simulink model "PowerSupplySimulation3"  (Simulink 8.6)
settings: Solver=VariableStepAuto  StartTime=0.0  StopTime=360e-6  RelTol=1e-3
values from neighbouring files (symbols this model uses):
  Ac = 1/(evalfr(G_ss, wcross)*evalfr(Gc1, wcross)*evalfr(Gc2, wcross))    [CurrentSourceController.m]    (also in VoltageSourceController.m)
  c2_val = 0.1e-6    (= 1e-07)    [VoltageSourceController.m]
  l1_val = 480e-8    (= 4.8e-06)    [CurrentSourceController.m]
  l2_val = 0.01e-6    (= 1e-08)    [VoltageSourceController.m]
  r_val = 1    [CurrentSourceController.m]
  rc2_val = 0.0001    [VoltageSourceController.m]
  rl1_val = 0.0002    [CurrentSourceController.m]
  rl2_val = 0.0001    [VoltageSourceController.m]
  Vd_val = 100    [CurrentSourceController.m]    (also in VoltageSourceController.m)
undefined symbols (not defined in the file or in its folder): den_c1, den_c2, num_c1, num_c2
libraries: powerlib x31, powerlib_meascontrol x2
settings Model: Creator=Akshay  LastModifiedBy=Akshay
settings SolverCC: ZeroCrossAlgorithm=Adaptive
settings DataIOCC: SaveFormat=Dataset  SignalLoggingSaveFormat=Dataset
settings OptimizationCC: ExpressionDepthLimit=128
settings DebuggingCC: UnderspecifiedInitializationDetection=Simplified  MergeDetectMultiDrivingBlocksExec=error  SolverPrmCheckMsg=none  FcnCallInpInsideContextMsg=EnableAllAsError  StateNameClashWarn=none
settings HardwareCC: ProdBitPerPointer=64  ProdLargestAtomicFloat=Float  ProdIntDivRoundTo=Zero  ProdEndianess=LittleEndian  ProdWordSize=64  ProdHWDeviceType=Intel->x86-64 (Windows64)
settings GRTTargetCC: GeneratePreprocessorConditionals=Use local settings  CombineOutputUpdateFcns=on  GRTInterface=off
settings ConfigComp: CovModelRefEnable=off

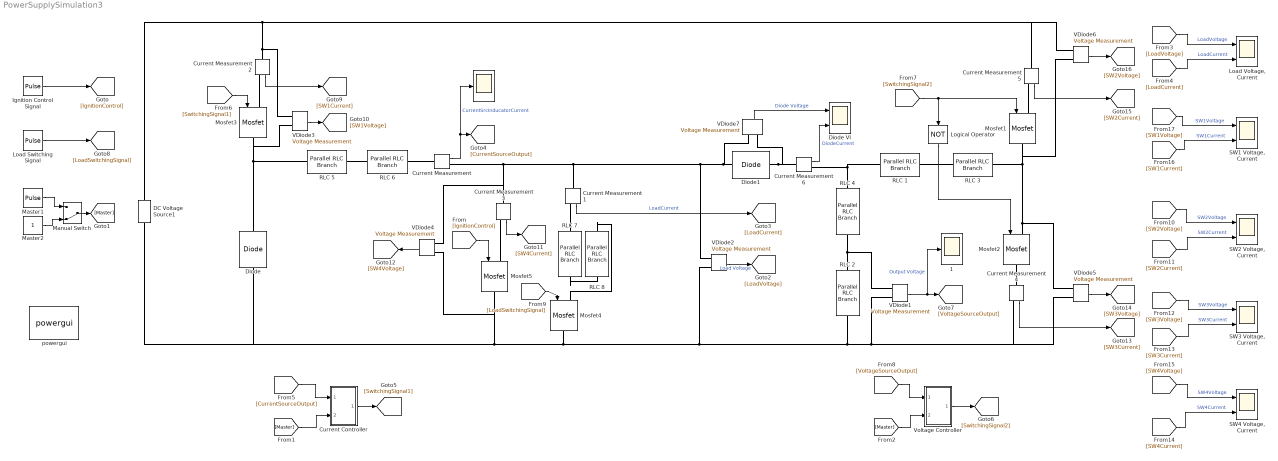
== system PowerSupplySimulation3 ==
  " " : Scope
  " 1" : Scope
  " RLC 1" : powerlib/Elements/Parallel RLC Branch  LConnTagsString=a  RConnTagsString=__new0  BranchType=R  Resistance=rl2_val  Inductance=5e-6  SetiL0=off  InitialCurrent=0  Capacitance=0.3e-6  Setx0=off  InitialVoltage=0  Measurements=None
  " RLC 2" : powerlib/Elements/Parallel RLC Branch  LConnTagsString=a  RConnTagsString=__new0  BranchType=C  Resistance=1  Inductance=1e-3  SetiL0=off  InitialCurrent=0  Capacitance=c2_val  Setx0=off  InitialVoltage=50  Measurements=None
  " RLC 3" : powerlib/Elements/Parallel RLC Branch  LConnTagsString=a  RConnTagsString=__new0  BranchType=L  Resistance=50  Inductance=l2_val  SetiL0=off  InitialCurrent=0  Capacitance=0.3e-6  Setx0=off  InitialVoltage=0  Measurements=None
  " RLC 4" : powerlib/Elements/Parallel RLC Branch  LConnTagsString=a  RConnTagsString=__new0  BranchType=R  Resistance=rc2_val  Inductance=1e-3  SetiL0=off  InitialCurrent=0  Capacitance=0.1e-6  Setx0=off  InitialVoltage=0  Measurements=None
  " RLC 5" : powerlib/Elements/Parallel RLC Branch  LConnTagsString=a  RConnTagsString=__new0  BranchType=R  Resistance=rl1_val  Inductance=5e-6  SetiL0=off  InitialCurrent=0  Capacitance=0.3e-6  Setx0=off  InitialVoltage=0  Measurements=None
  " RLC 6" : powerlib/Elements/Parallel RLC Branch  LConnTagsString=a  RConnTagsString=__new0  BranchType=L  Resistance=50  Inductance=l1_val  SetiL0=off  InitialCurrent=100  Capacitance=0.3e-6  Setx0=off  InitialVoltage=0  Measurements=None
  " RLC 7" : powerlib/Elements/Parallel RLC Branch  LConnTagsString=a  RConnTagsString=__new0  BranchType=R  Resistance=r_val  Inductance=1e-3  SetiL0=off  InitialCurrent=0  Capacitance=0.1e-6  Setx0=off  InitialVoltage=0  Measurements=None
  " RLC 8" : powerlib/Elements/Parallel RLC Branch  LConnTagsString=a  RConnTagsString=__new0  BranchType=L  Resistance=r_val  Inductance=15e-6  SetiL0=off  InitialCurrent=0  Capacitance=0.1e-6  Setx0=off  InitialVoltage=0  Measurements=None
  Current Measurement{,1..6} (7 alike) : powerlib/Measurements/Current Measurement  PhasorSimulation=off  OutputType=Complex  PSBequivalent=0
  Current Controller : Subsystem
  DC Voltage Source1 : powerlib/Electrical Sources/DC Voltage Source  Amplitude=Vd_val  Measurements=Voltage
  Diode : powerlib/Power Electronics/Diode  Ron=0.001  Lon=0  Vf=0.8  IC=0  UseSnubber=off  Rs=500  Cs=250e-9  Measurements=off
  Diode VI : Scope  NumInputPorts=2
  Diode1 : powerlib/Power Electronics/Diode  Ron=0.001  Lon=0  Vf=0.8  IC=0  UseSnubber=off  Rs=500  Cs=250e-9  Measurements=off
  Ignition Control Signal : DiscretePulseGenerator  PulseType=Time based  Period=180e-6  PulseWidth=94  PhaseDelay=6*1.8e-6
  Load Switching Signal : DiscretePulseGenerator  PulseType=Time based  Period=180e-6  PulseWidth=5  PhaseDelay=1.8e-6
  "Load Voltage, Current" : Scope  NumInputPorts=2
  Logical Operator : Logic  Operator=NOT  AllPortsSameDT=off  OutDataTypeStr=boolean
  Manual Switch : ManualSwitch  CurrentSetting=0
  Master1 : DiscretePulseGenerator  PulseType=Time based  Period=180e-6  PulseWidth=6
  Master2 : Constant
  Mosfet{1..5} (5 alike) : powerlib/Power Electronics/Mosfet  Ron=0.00001  Lon=0  Rd=0.0000000000001  Vfd=0  IC=0  Rs=1e5  Cs=inf  Measurements=off
  "SW1 Voltage, Current" : Scope  NumInputPorts=2
  "SW2 Voltage, Current" : Scope  NumInputPorts=2
  "SW3 Voltage, Current" : Scope  NumInputPorts=2
  "SW4 Voltage, Current" : Scope  NumInputPorts=2
  VDiode{1..7} (7 alike) : powerlib/Measurements/Voltage Measurement  PhasorSimulation=off  OutputType=Complex  PSBequivalent=0
  Voltage Controller : Subsystem
  powergui : powerlib/powergui  Priority=1  SimulationMode=Continuous  SolverType=Backward Euler  SampleTime=5e-07  frequency=60  SPID=on  DisableSnubberDevices=off  DisableRonSwitches=off  DisableVfSwitches=off  SwTol=0  DisplayEquations=off  Interpol=off  ExternalGateDelay=off  methode=off  Ts=0  FunctionMessages=off  echomessages=off  HookPort=off  EnableUseOfTLC=off  x0status=zero  frequencyindice=0  Pbase=100e6  ErrMax=1e-4  Iterations=50  UnitsV=kV  UnitsW=MW  buscounter=0  RestoreLinks=warning  ResistiveCurrentMeasurement=off  Frange=[0:2:500]  Ylog=off  Xlog=on  ShowGrid=off  save=off  variable=ZData  structure=ScopeData  ZoomFFT=off  StartTime=0.0  cycles=5  DisplayStyle=2  fundamental=50  FreqAxis=off  MaxFrequency=50000  frequencyindicesteady=1  RmsSteady=1  display=off
  wires:
  Logical Operator/1 -> Mosfet2/1
  VDiode1/1 -> " 1"/1, [VoltageSourceOutput]  "Output Voltage"
  Ignition Control Signal/1 -> [IgnitionControl]
  [IgnitionControl] -> Mosfet5/1
  VDiode2/1 -> [LoadVoltage]  "Load Voltage"
  Current Measurement1/1 -> [LoadCurrent]  "LoadCurrent"
  [LoadVoltage] -> "Load Voltage, Current"/1  "LoadVoltage"
  [LoadCurrent] -> "Load Voltage, Current"/2  "LoadCurrent"
  Current Measurement/1 -> " "/1, [CurrentSourceOutput]  "CurrentSrcInducatorCurrent"
  [SwitchingSignal1] -> Mosfet3/1
  [SwitchingSignal2] -> Logical Operator/1, Mosfet1/1
  Load Switching Signal/1 -> [LoadSwitchingSignal]
  [LoadSwitchingSignal] -> Mosfet4/1
  Manual Switch/1 -> [Master]
  Master1/1 -> Manual Switch/1
  Master2/1 -> Manual Switch/2
  [CurrentSourceOutput] -> Current Controller/1(Inductor Current)
  [Master] -> Current Controller/2(In2)
  Current Controller/1(Duty1) -> [SwitchingSignal1]
  [VoltageSourceOutput] -> Voltage Controller/1(In1)
  [Master] -> Voltage Controller/2(In2)
  Voltage Controller/1(Out1) -> [SwitchingSignal2]
  Current Measurement2/1 -> [SW1Current]
  VDiode3/1 -> [SW1Voltage]
  Current Measurement3/1 -> [SW4Current]
  VDiode4/1 -> [SW4Voltage]
  Current Measurement4/1 -> [SW3Current]
  VDiode5/1 -> [SW3Voltage]
  VDiode6/1 -> [SW2Voltage]
  Current Measurement5/1 -> [SW2Current]
  [SW2Voltage] -> "SW2 Voltage, Current"/1  "SW2Voltage"
  [SW2Current] -> "SW2 Voltage, Current"/2  "SW2Current"
  [SW3Voltage] -> "SW3 Voltage, Current"/1  "SW3Voltage"
  [SW3Current] -> "SW3 Voltage, Current"/2  "SW3Current"
  [SW1Voltage] -> "SW1 Voltage, Current"/1  "SW1Voltage"
  [SW1Current] -> "SW1 Voltage, Current"/2  "SW1Current"
  [SW4Voltage] -> "SW4 Voltage, Current"/1  "SW4Voltage"
  [SW4Current] -> "SW4 Voltage, Current"/2  "SW4Current"
  VDiode7/1 -> Diode VI/1  "Diode Voltage"
  Current Measurement6/1 -> Diode VI/2  "DiodeCurrent"
  connections:
  " RLC 3"/RConn1 -- Mosfet1/RConn1 -- VDiode6/LConn2 -- VDiode5/LConn1 -- Mosfet2/LConn1
  " RLC 2"/RConn1 -- VDiode4/LConn1 -- Mosfet5/RConn1 -- DC Voltage Source1/LConn1 -- Diode/LConn1 -- Mosfet4/RConn1 -- VDiode2/LConn2 -- Current Measurement4/RConn1 -- VDiode5/LConn2 -- VDiode1/LConn2
  " RLC 2"/LConn1 -- " RLC 4"/RConn1 -- VDiode1/LConn1
  " RLC 1"/RConn1 -- " RLC 3"/LConn1
  " RLC 5"/LConn1 -- VDiode3/LConn2 -- Mosfet3/RConn1 -- Diode/RConn1
  DC Voltage Source1/RConn1 -- Current Measurement5/LConn1 -- VDiode6/LConn1 -- VDiode3/LConn1 -- Current Measurement2/LConn1
  " RLC 5"/RConn1 -- " RLC 6"/LConn1
  Current Measurement/LConn1 -- " RLC 6"/RConn1
  Current Measurement1/RConn1 -- " RLC 7"/LConn1
  Current Measurement2/RConn1 -- Mosfet3/LConn1
  Current Measurement3/RConn1 -- Mosfet5/LConn1
  Current Measurement4/LConn1 -- Mosfet2/RConn1
  Current Measurement5/RConn1 -- Mosfet1/LConn1
  " RLC 7"/RConn1 -- " RLC 8"/RConn1
  " RLC 8"/LConn1 -- Mosfet4/LConn1
  VDiode2/LConn1 -- Current Measurement1/LConn1 -- VDiode4/LConn2 -- Current Measurement3/LConn1 -- Current Measurement/RConn1 -- VDiode7/LConn1 -- Diode1/LConn1
  Diode1/RConn1 -- Current Measurement6/LConn1 -- VDiode7/LConn2
  " RLC 4"/LConn1 -- " RLC 1"/LConn1 -- Current Measurement6/RConn1

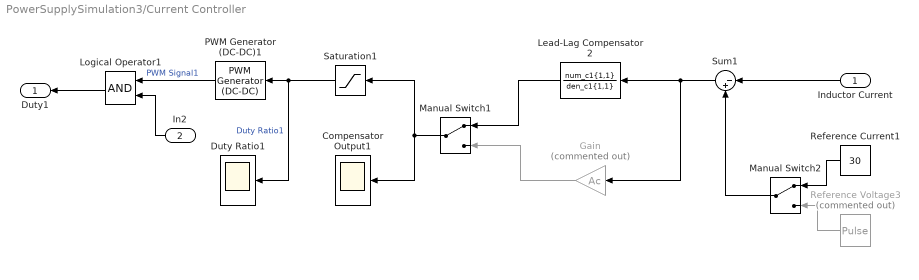
== system PowerSupplySimulation3/Current Controller ==
  Inductor Current : Inport
  In2 : Inport  Port=2
  Compensator Output1 : Scope
  Duty Ratio1 : Scope
  Gain : Gain  Commented=on  Gain=Ac
  Lead-Lag Compensator2 : TransferFcn  Numerator=num_c1{1,1}  Denominator=den_c1{1,1}
  Logical Operator1 : Logic  AllPortsSameDT=off  OutDataTypeStr=boolean
  Manual Switch1 : ManualSwitch
  Manual Switch2 : ManualSwitch
  PWM Generator (DC-DC)1 : powerlib_meascontrol/Pulse & Signal Generators/PWM Generator (DC-DC)  Fsw=1e6  Ts=0
  Reference Current1 : Constant  Value=30
  Reference Voltage3 : DiscretePulseGenerator  Commented=on  PulseType=Time based  Amplitude=70  Period=180e-6  PulseWidth=6
  Saturation1 : Saturate  UpperLimit=1  LowerLimit=0  ZeroCross=off
  Sum1 : Sum  Inputs=|-+
  Duty1 : Outport
  wires:
  In2/1 -> Logical Operator1/2
  Logical Operator1/1 -> Duty1/1
  Lead-Lag Compensator2/1 -> Manual Switch1/1
  Saturation1/1 -> Duty Ratio1/1, PWM Generator (DC-DC)1/1  "Duty Ratio1"
  Inductor Current/1 -> Sum1/1
  PWM Generator (DC-DC)1/1 -> Logical Operator1/1  "PWM Signal1"
  Manual Switch2/1 -> Sum1/2
  Reference Voltage3/1 -> Manual Switch2/2
  Manual Switch1/1 -> Compensator Output1/1, Saturation1/1
  Sum1/1 -> Gain/1, Lead-Lag Compensator2/1
  Reference Current1/1 -> Manual Switch2/1
  Gain/1 -> Manual Switch1/2

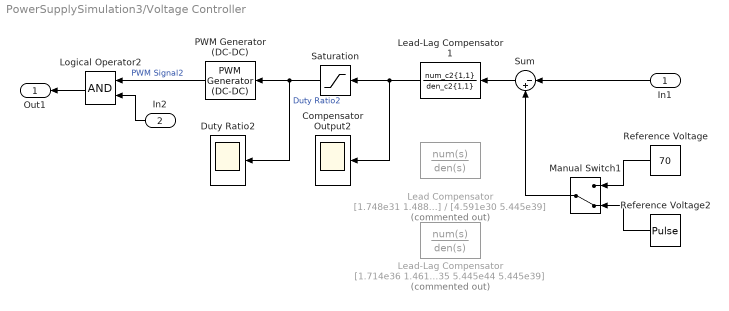
== system PowerSupplySimulation3/Voltage Controller ==
  In1 : Inport
  In2 : Inport  Port=2
  Compensator Output2 : Scope
  Duty Ratio2 : Scope
  Lead Compensator : TransferFcn  Commented=on  Numerator=[1.748e31 1.488e39]  Denominator=[4.591e30 5.445e39]
  Lead-Lag Compensator : TransferFcn  Commented=on  Numerator=[1.714e36 1.461e44 1.459e49]  Denominator=[4.591e35 5.445e44 5.445e39]
  Lead-Lag Compensator1 : TransferFcn  Numerator=num_c2{1,1}  Denominator=den_c2{1,1}
  Logical Operator2 : Logic  AllPortsSameDT=off  OutDataTypeStr=boolean
  Manual Switch1 : ManualSwitch  CurrentSetting=0
  PWM Generator (DC-DC) : powerlib_meascontrol/Pulse & Signal Generators/PWM Generator (DC-DC)  Fsw=1e6  Ts=0
  Reference Voltage : Constant  Value=70
  Reference Voltage2 : DiscretePulseGenerator  PulseType=Time based  Amplitude=70  Period=180e-6  PulseWidth=7  PhaseDelay=-1e-6
  Saturation : Saturate  UpperLimit=1  LowerLimit=0  ZeroCross=off
  Sum : Sum  Inputs=|-+
  Out1 : Outport
  wires:
  Logical Operator2/1 -> Out1/1
  Lead-Lag Compensator1/1 -> Compensator Output2/1, Saturation/1
  Saturation/1 -> Duty Ratio2/1, PWM Generator (DC-DC)/1  "Duty Ratio2"
  Sum/1 -> Lead-Lag Compensator1/1
  In2/1 -> Logical Operator2/2
  PWM Generator (DC-DC)/1 -> Logical Operator2/1  "PWM Signal2"
  In1/1 -> Sum/1
  Reference Voltage/1 -> Manual Switch1/1
  Manual Switch1/1 -> Sum/2
  Reference Voltage2/1 -> Manual Switch1/2
